simulink subsystem "rss_MotoSpdHiLvl1Dia"  (R2023a)
settings: Solver=VariableStepAuto  StartTime=0.0  StopTime=10.0  RelTol=1e-3
undefined symbols (not defined in the file): Cdbl_nElecAgSpdMaxVal, ENM_TYPE_FALT, Gu16_ctMotoSpdHiLvl1ConfCnt_C, Gu16_ctMotoSpdHiLvl1RcvyCnt_C, Gu16_nMotoSpdHiLvl1ConfTrs_C, Gu16_nMotoSpdHiLvl1RcvyTrs_C
libraries: vhit_control_library x1, lib_fault_definiteness x1
settings Model: Creator=xiaoqiang.yuan  LastModifiedBy=xiaoqiang.yuan

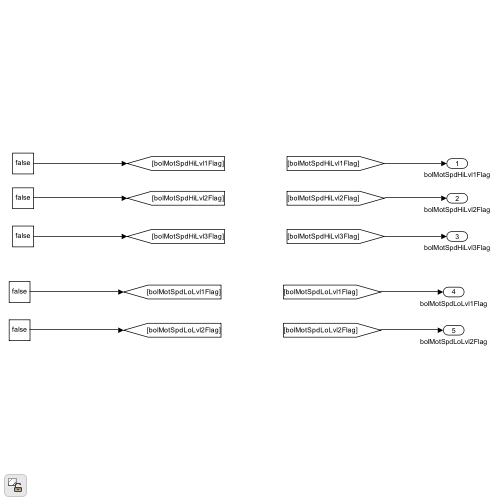
[thumbnail: Simulink's stored preview of the top-level diagram]
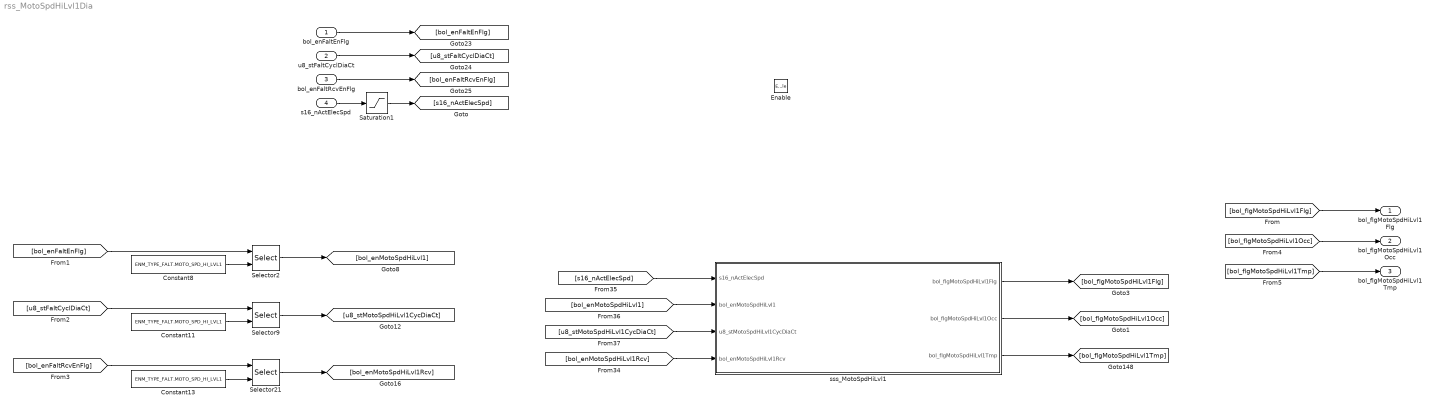
== system rss_MotoSpdHiLvl1Dia ==
  bol_enFaltEnFlg : Inport  OutDataTypeStr=boolean
  u8_stFaltCyclDiaCt : Inport  Port=2  OutDataTypeStr=uint8
  bol_enFaltRcvEnFlg : Inport  Port=3  OutDataTypeStr=boolean
  s16_nActElecSpd : Inport  Port=4  OutDataTypeStr=dt_Standardize_s16p15b0
  Enable : EnablePort
  Constant11 : Constant  Value=ENM_TYPE_FALT.MOTO_SPD_HI_LVL1
  Constant13 : Constant  Value=ENM_TYPE_FALT.MOTO_SPD_HI_LVL1
  Constant8 : Constant  Value=ENM_TYPE_FALT.MOTO_SPD_HI_LVL1
  Saturation1 : Saturate  UpperLimit=Cdbl_nElecAgSpdMaxVal  LowerLimit=-Cdbl_nElecAgSpdMaxVal
  Selector2 : Selector  IndexMode=Zero-based  InputPortWidth=Cdbl_numFaltDiaNum  IndexOptions=Index vector (port)  Indices=[1 3]  OutputSizes=1
  Selector21 : Selector  IndexMode=Zero-based  InputPortWidth=Cdbl_numFaltDiaNum  IndexOptions=Index vector (port)  Indices=[1 3]  OutputSizes=1
  Selector9 : Selector  IndexMode=Zero-based  InputPortWidth=Cdbl_numFaltDiaNum  IndexOptions=Index vector (port)  Indices=[1 3]  OutputSizes=1
  sss_MotoSpdHiLvl1 : Subsystem
  bol_flgMotoSpdHiLvl1Flg : Outport  OutDataTypeStr=boolean
  bol_flgMotoSpdHiLvl1Occ : Outport  Port=2  OutDataTypeStr=boolean
  bol_flgMotoSpdHiLvl1Tmp : Outport  Port=3  OutDataTypeStr=boolean
  wires:
  Selector9/1 -> [u8_stMotoSpdHiLvl1CycDiaCt]
  [bol_enMotoSpdHiLvl1Rcv] -> sss_MotoSpdHiLvl1/4(bol_enMotoSpdHiLvl1Rcv)
  [bol_enFaltEnFlg] -> Selector2/1
  Selector2/1 -> [bol_enMotoSpdHiLvl1]
  Constant11/1 -> Selector9/2
  Constant13/1 -> Selector21/2
  Selector21/1 -> [bol_enMotoSpdHiLvl1Rcv]
  sss_MotoSpdHiLvl1/2(bol_flgMotoSpdHiLvl1Occ) -> [bol_flgMotoSpdHiLvl1Occ]
  Constant8/1 -> Selector2/2
  [u8_stMotoSpdHiLvl1CycDiaCt] -> sss_MotoSpdHiLvl1/3(u8_stMotoSpdHiLvl1CycDiaCt)
  s16_nActElecSpd/1 -> Saturation1/1
  [bol_enFaltRcvEnFlg] -> Selector21/1
  [bol_flgMotoSpdHiLvl1Occ] -> bol_flgMotoSpdHiLvl1Occ/1
  [u8_stFaltCyclDiaCt] -> Selector9/1
  [bol_enMotoSpdHiLvl1] -> sss_MotoSpdHiLvl1/2(bol_enMotoSpdHiLvl1)
  u8_stFaltCyclDiaCt/1 -> [u8_stFaltCyclDiaCt]
  [bol_flgMotoSpdHiLvl1Flg] -> bol_flgMotoSpdHiLvl1Flg/1
  Saturation1/1 -> [s16_nActElecSpd]
  bol_enFaltRcvEnFlg/1 -> [bol_enFaltRcvEnFlg]
  bol_enFaltEnFlg/1 -> [bol_enFaltEnFlg]
  sss_MotoSpdHiLvl1/1(bol_flgMotoSpdHiLvl1Flg) -> [bol_flgMotoSpdHiLvl1Flg]
  [s16_nActElecSpd] -> sss_MotoSpdHiLvl1/1(s16_nActElecSpd)
  [bol_flgMotoSpdHiLvl1Tmp] -> bol_flgMotoSpdHiLvl1Tmp/1
  sss_MotoSpdHiLvl1/3(bol_flgMotoSpdHiLvl1Tmp) -> [bol_flgMotoSpdHiLvl1Tmp]

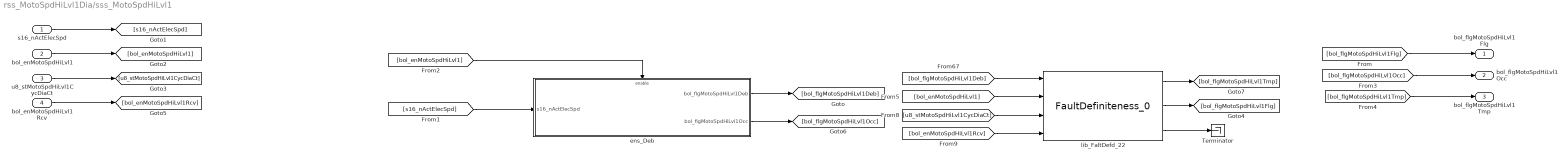
== system rss_MotoSpdHiLvl1Dia/sss_MotoSpdHiLvl1 ==
  s16_nActElecSpd : Inport
  bol_enMotoSpdHiLvl1 : Inport  Port=2
  u8_stMotoSpdHiLvl1CycDiaCt : Inport  Port=3
  bol_enMotoSpdHiLvl1Rcv : Inport  Port=4
  Terminator : Terminator
  ens_Deb : Subsystem
  lib_FaltDefd_22 : lib_fault_definiteness/FaultDefiniteness_0  lb_FaltWaitRecvCnt=Gu16_ctMotoSpdHiLvl1ConfCnt_C
  bol_flgMotoSpdHiLvl1Flg : Outport
  bol_flgMotoSpdHiLvl1Occ : Outport  Port=2
  bol_flgMotoSpdHiLvl1Tmp : Outport  Port=3
  wires:
  [bol_flgMotoSpdHiLvl1Tmp] -> bol_flgMotoSpdHiLvl1Tmp/1
  u8_stMotoSpdHiLvl1CycDiaCt/1 -> [u8_stMotoSpdHiLvl1CycDiaCt]
  [bol_flgMotoSpdHiLvl1Occ] -> bol_flgMotoSpdHiLvl1Occ/1
  [bol_flgMotoSpdHiLvl1Deb] -> lib_FaltDefd_22/1
  [s16_nActElecSpd] -> ens_Deb/1(s16_nActElecSpd)
  bol_enMotoSpdHiLvl1/1 -> [bol_enMotoSpdHiLvl1]
  [u8_stMotoSpdHiLvl1CycDiaCt] -> lib_FaltDefd_22/3
  [bol_enMotoSpdHiLvl1Rcv] -> lib_FaltDefd_22/4
  ens_Deb/2(bol_flgMotoSpdHiLvl1Occ) -> [bol_flgMotoSpdHiLvl1Occ]
  lib_FaltDefd_22/3 -> Terminator/1
  [bol_flgMotoSpdHiLvl1Flg] -> bol_flgMotoSpdHiLvl1Flg/1
  [bol_enMotoSpdHiLvl1] -> lib_FaltDefd_22/2
  s16_nActElecSpd/1 -> [s16_nActElecSpd]
  bol_enMotoSpdHiLvl1Rcv/1 -> [bol_enMotoSpdHiLvl1Rcv]
  [bol_enMotoSpdHiLvl1] -> ens_Deb/Enable
  ens_Deb/1(bol_flgMotoSpdHiLvl1Deb) -> [bol_flgMotoSpdHiLvl1Deb]
  lib_FaltDefd_22/2 -> [bol_flgMotoSpdHiLvl1Flg]
  lib_FaltDefd_22/1 -> [bol_flgMotoSpdHiLvl1Tmp]

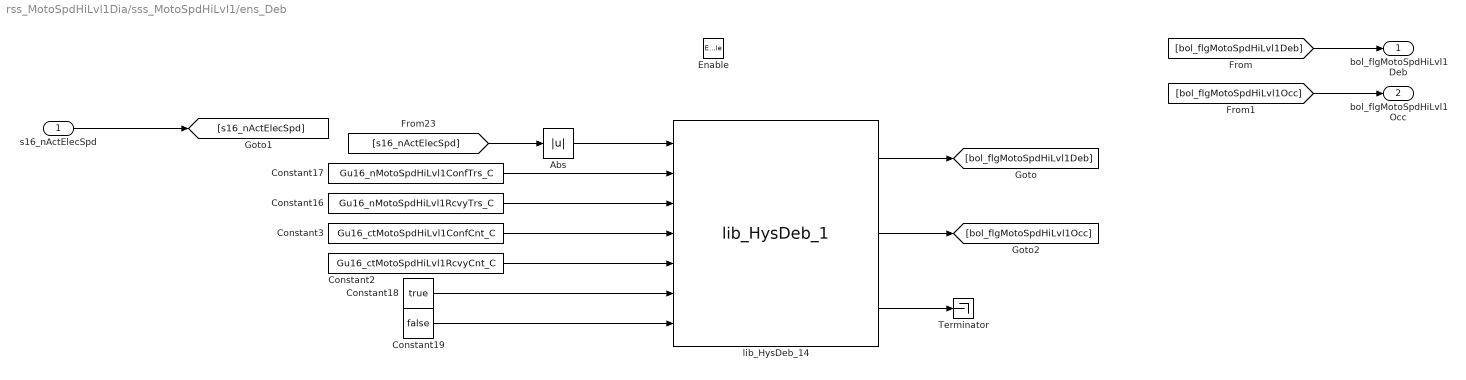
== system rss_MotoSpdHiLvl1Dia/sss_MotoSpdHiLvl1/ens_Deb ==
  s16_nActElecSpd : Inport
  Enable : EnablePort
  Abs : Abs  SaturateOnIntegerOverflow=off
  Constant16 : Constant  Value=Gu16_nMotoSpdHiLvl1RcvyTrs_C
  Constant17 : Constant  Value=Gu16_nMotoSpdHiLvl1ConfTrs_C
  Constant18 : Constant  Value=true  OutDataTypeStr=boolean
  Constant19 : Constant  Value=false  OutDataTypeStr=boolean
  Constant2 : Constant  Value=Gu16_ctMotoSpdHiLvl1RcvyCnt_C
  Constant3 : Constant  Value=Gu16_ctMotoSpdHiLvl1ConfCnt_C
  Terminator : Terminator
  lib_HysDeb_14 : vhit_control_library/lib_HysDeb_1  lb_parInitOutp=0
  bol_flgMotoSpdHiLvl1Deb : Outport
  bol_flgMotoSpdHiLvl1Occ : Outport  Port=2
  wires:
  Abs/1 -> lib_HysDeb_14/1
  Constant2/1 -> lib_HysDeb_14/5
  Constant3/1 -> lib_HysDeb_14/4
  Constant16/1 -> lib_HysDeb_14/3
  Constant17/1 -> lib_HysDeb_14/2
  [bol_flgMotoSpdHiLvl1Occ] -> bol_flgMotoSpdHiLvl1Occ/1
  lib_HysDeb_14/3 -> Terminator/1
  lib_HysDeb_14/2 -> [bol_flgMotoSpdHiLvl1Occ]
  Constant19/1 -> lib_HysDeb_14/7
  Constant18/1 -> lib_HysDeb_14/6
  [s16_nActElecSpd] -> Abs/1
  s16_nActElecSpd/1 -> [s16_nActElecSpd]
  [bol_flgMotoSpdHiLvl1Deb] -> bol_flgMotoSpdHiLvl1Deb/1
  lib_HysDeb_14/1 -> [bol_flgMotoSpdHiLvl1Deb]
